simulink model "QUESTION3"  (R2021b)
settings: Solver=VariableStepAuto  StartTime=0.0  StopTime=200  RelTol=1e-3
settings Model: Creator=Progg  LastModifiedBy=Progg

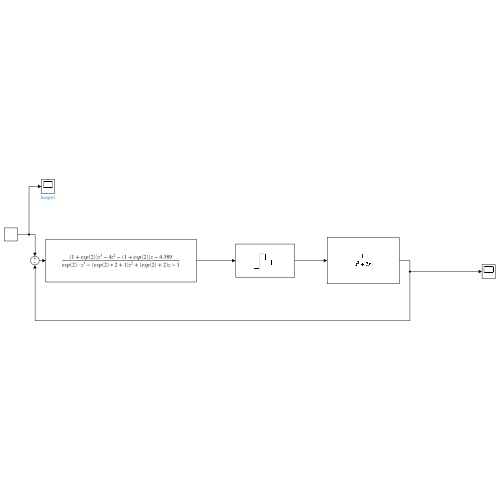
[thumbnail: Simulink's stored preview of the top-level diagram]
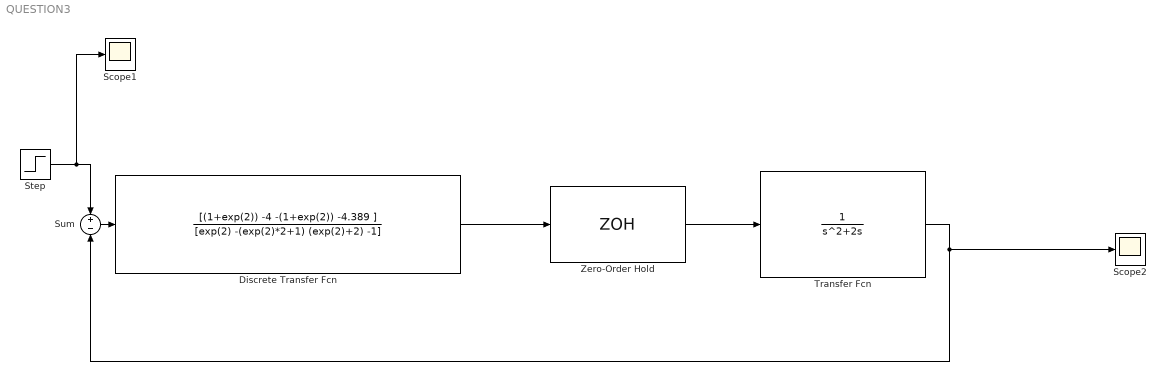
== system QUESTION3 ==
  Discrete Transfer Fcn : DiscreteTransferFcn  Numerator=[(1+exp(2)) -4 -(1+exp(2)) -4.389 ]  Denominator=[exp(2) -(exp(2)*2+1) (exp(2)+2) -1]
  Scope1 : Scope
  Scope2 : Scope
  Step : Step  SampleTime=0
  Sum : Sum  Inputs=+-
  Transfer Fcn : TransferFcn  Denominator=[1 2 0]
  Zero-Order Hold : ZeroOrderHold  SampleTime=-1
  wires:
  Discrete Transfer Fcn/1 -> Zero-Order Hold/1
  Zero-Order Hold/1 -> Transfer Fcn/1
  Step/1 -> Scope1/1, Sum/1
  Transfer Fcn/1 -> Scope2/1, Sum/2
  Sum/1 -> Discrete Transfer Fcn/1
